simulink model "GS_LQI_s_v_seno_function"  (R2023b)
settings: Solver=VariableStepAuto  StartTime=0.0  StopTime=10.0  RelTol=1e-7
undefined symbols (not defined in the file or in its folder): Disturbo
settings Model: Creator=giova  LastModifiedBy=miche

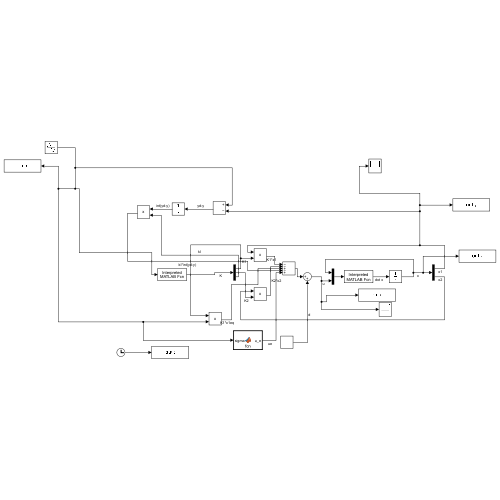
[thumbnail: Simulink's stored preview of the top-level diagram]
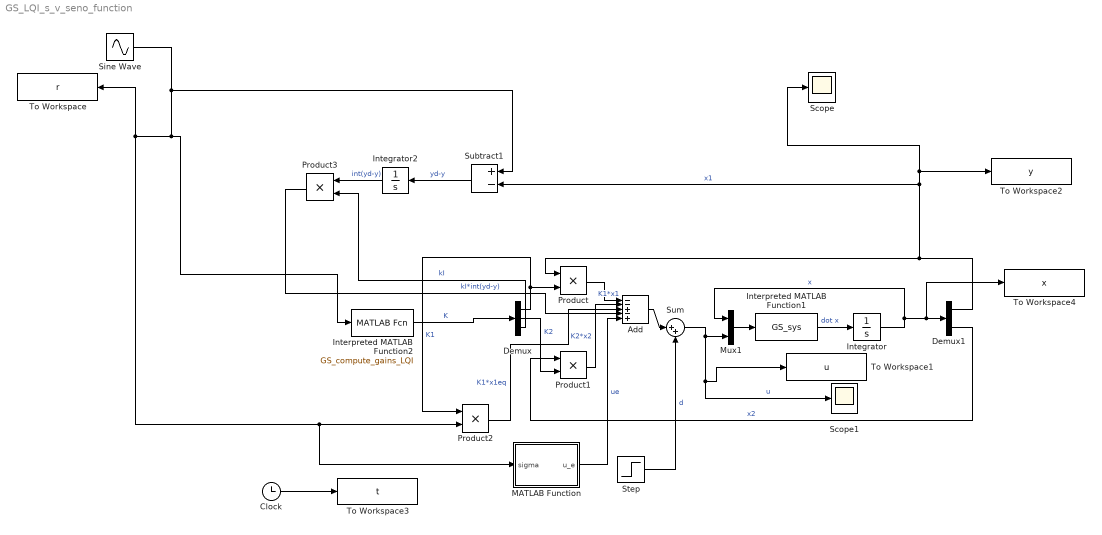
== system GS_LQI_s_v_seno_function ==
  Add : Sum  Inputs=--+-+
  Clock : Clock
  Demux : Demux  Outputs=3
  Demux1 : Demux  Outputs=2
  Integrator : Integrator
  Integrator2 : Integrator
  Interpreted MATLAB Function1 : MATLABFcn  MATLABFcn=GS_sys  OutputDimensions=2
  Interpreted MATLAB Function2 : MATLABFcn  MATLABFcn=GS_compute_gains_LQI  OutputDimensions=3
  MATLAB Function : MATLAB Function  TreatAsAtomicUnit=on
  Mux1 : Mux  Inputs=2
  Product{,1..3} (4 alike) : Product
  Scope : Scope
  Scope1 : Scope
  Sine Wave : Sin  Amplitude=3.14  SampleTime=0
  Step : Step  Time=5  After=Disturbo  SampleTime=0
  Subtract1 : Sum  Inputs=+-
  Sum : Sum  Inputs=|++
  To Workspace : ToWorkspace  VariableName=r  SampleTime=-1
  To Workspace1 : ToWorkspace  VariableName=u  SampleTime=-1
  To Workspace2 : ToWorkspace  VariableName=y  SampleTime=-1
  To Workspace3 : ToWorkspace  VariableName=t  SampleTime=-1
  To Workspace4 : ToWorkspace  VariableName=x  SampleTime=-1
  wires:
  Interpreted MATLAB Function1/1 -> Integrator/1  "dot x"
  Sine Wave/1 -> MATLAB Function/1(sigma), Product2/2, To Workspace/1, Interpreted MATLAB Function2/1, Subtract1/1
  Product3/1 -> Add/4  "kI*int(yd-y)"
  Demux/3 -> Product3/2  "kI"
  Add/1 -> Sum/1
  Mux1/1 -> Interpreted MATLAB Function1/1
  Product1/1 -> Add/2  "K2*x2"
  Demux/2 -> Product1/2  "K2"
  Clock/1 -> To Workspace3/1
  Demux1/1 -> Product/1, Scope/1, To Workspace2/1, Subtract1/2  "x1"
  Integrator/1 -> To Workspace4/1, Demux1/1, Mux1/1  "x"
  Integrator2/1 -> Product3/1  "int(yd-y)"
  Interpreted MATLAB Function2/1 -> Demux/1  "K"
  Demux/1 -> Product2/1, Product/2  "K1"
  Sum/1 -> Mux1/2, To Workspace1/1, Scope1/1  "u"
  Step/1 -> Sum/2  "d"
  Product/1 -> Add/1  "K1*x1"
  Subtract1/1 -> Integrator2/1  "yd-y"
  Demux1/2 -> Product1/1  "x2"
  Product2/1 -> Add/3  "K1*x1eq"
  MATLAB Function/1(u_e) -> Add/5  "ue"

== matlab function GS_LQI_s_v_seno_function/MATLAB Function ==
  data: sigma input; u_e output
function u_e = fcn(sigma)

u_e=9.81*sin(sigma);
